simulink model "pendulo_invertido"  (R2025a)
settings: Solver=VariableStepAuto  StartTime=0.0  StopTime=10  RelTol=1e-3

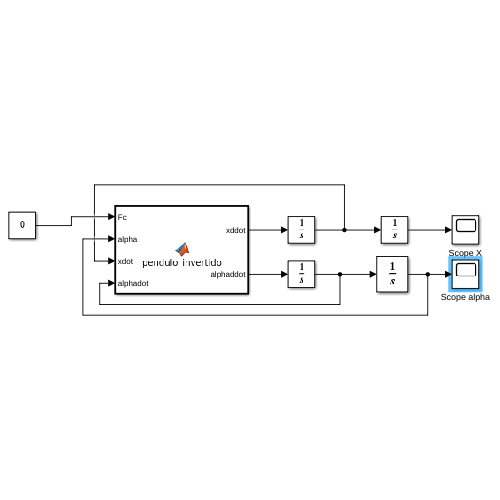
[thumbnail: Simulink's stored preview of the top-level diagram]
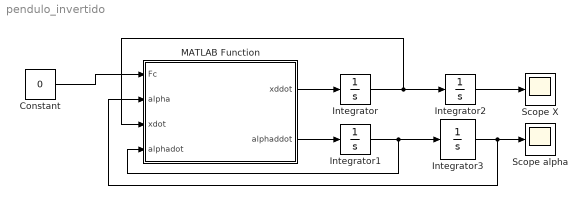
== system pendulo_invertido ==
  Constant : Constant  Value=0
  Integrator : Integrator
  Integrator1 : Integrator
  Integrator2 : Integrator
  Integrator3 : Integrator  InitialCondition=pi/180
  MATLAB Function : MATLAB Function  TreatAsAtomicUnit=on
  Scope X : Scope
      settings: ActiveDisplayYMinimum=-0.37734415005753752  ActiveDisplayYMaximum=0.46377100485462031
  Scope alpha : Scope
      settings: ActiveDisplayYMinimum=-64.7197994486354  ActiveDisplayYMaximum=167.47947197886282
  wires:
  MATLAB Function/1(xddot) -> Integrator/1
  Constant/1 -> MATLAB Function/1(Fc)
  Integrator/1 -> MATLAB Function/3(xdot), Integrator2/1
  MATLAB Function/2(alphaddot) -> Integrator1/1
  Integrator1/1 -> MATLAB Function/4(alphadot), Integrator3/1
  Integrator2/1 -> Scope X/1
  Integrator3/1 -> MATLAB Function/2(alpha), Scope alpha/1

== matlab function pendulo_invertido/MATLAB Function ==
  data: Fc input; alpha input; xdot input; alphadot input; xddot output; alphaddot output
function [xddot, alphaddot] = pendulo_invertido(Fc, alpha, xdot, alphadot)
    % Parámetros físicos
    Ip  = 0.0079;      % kg*m^2
    Mc  = 0.7031;      % kg
    lp  = 0.3302;      % m
    Mp  = 0.23;        % kg
    Beq = 4.3;         % N*s/m
    g   = 9.81;        % m/s^2
    Bp  = 0.0024;      % N*s/rad

    % Denominador común
    denominador = (Mc + Mp)*Ip + Mc*Mp*lp^2 + (Mp^2 * lp^2 * (sin(alpha))^2);

    % Aceleración del carro
    xddot = ((Ip + Mp*lp^2)*Fc ...
            + Mp^2*lp^2*g*cos(alpha)*sin(alpha) ...
            - (Ip + Mp*lp^2)*Beq*xdot ...
            - (Ip*Mp*lp - Mp^2*lp^3)*(alphadot^2)*sin(alpha) ...
            - Mp*lp*alphadot*Bp*cos(alpha)) / denominador;

    % Aceleración angular del péndulo
    alphaddot = ((Mc + Mp)*Mp*g*lp*sin(alpha) ...
                - (Mc + Mp)*Bp*alphadot ...
                + Fc*Mp*lp*cos(alpha) ...
                - Mp^2*lp^2*(alphadot^2)*sin(alpha)*cos(alpha) ...
                - Beq*Mp*lp*xdot*cos(alpha)) / denominador;
end
